simulink model "ScpAp_SafetyModeManager"  (R2025b)
settings: Solver=FixedStepDiscrete  StartTime=0.0  StopTime=10.0  FixedStep=0.02  RelTol=1e-3
undefined symbols (not defined in the file): SafetyMode_L2p_IDT, VechSafetyStatus_L2p_IDT
settings Model: DataDictionary=EgasPOC.sldd  Creator=IAST283  LastModifiedBy=IAST283
settings DataIOCC: SaveFormat=StructureWithTime
settings OptimizationCC: DefaultParameterBehavior=Inlined  EnhancedBackFolding=on  PassReuseOutputArgsAs=Individual arguments  ZeroExternalMemoryAtStartup=off  ZeroInternalMemoryAtStartup=off  OptimizeBlockOrder=speed  DifferentSizesBufferReuse=on  OptimizationCustomize=off  EfficientTunableParamExpr=on
settings DebuggingCC: ParameterTunabilityLossMsg=error
settings SFSimCC: MATLABDynamicMemAlloc=off
settings RTWCC: SystemTargetFile=autosar.tlc  GenCodeOnly=on  TemplateMakefile=ert_default_tmf  DataTypeReplacement=CDataTypesFixedWidth  Description=AUTOSAR
settings CodeAppCC: ForceParamTrailComments=on  IgnoreCustomStorageClasses=off  OperatorAnnotations=on  SimulinkDataObjDesc=on  SFDataObjDesc=on  InsertBlockDesc=on
settings STFCustomTargetCC: SystemTargetFile=autosar.tlc  TargetLangStandard=C99 (ISO)  MultiwordLength=256.0  ParMdlRefBuildCompliant=on  CompOptLevelCompliant=on  ConcurrentExecutionCompliant=off  IncludeMdlTerminateFcn=off  CombineOutputUpdateFcns=on  SuppressErrorStatus=on  ERTCustomFileBanners=on  SupportNonFinite=off  SupportComplex=off  SupportContinuousTime=off  SupportNonInlinedSFcns=off  RemoveResetFunc=on  MATLABClassNameForMDSCustomization=Simulink.SoftwareTarget.ERTCustomization  AutosarCompliant=on  GRTInterface=off  UseToolchainInfoCompliant=on  LookupTableObjectStructAxisOrder=2,1,3,4,...  LUTObjectStructOrderEvenSpacing=Size,Table,Breakpoints  AutosarMatrixIOAsArray=off  AutosarSchemaVersion=R20-11  AutosarCompilerAbstraction=off  DisableAUTOSARRoutinesHostLibrary=off  AutosarMaxShortNameLength=128.0
settings ERTTargetCC: ERTCustomFileTemplate=example_file_process.tlc  BooleanTrueId=TRUE  BooleanFalseId=FALSE  TargetLangStandard=C99 (ISO)  ConcurrentExecutionCompliant=off  IncludeMdlTerminateFcn=off  SuppressErrorStatus=on  SupportNonFinite=off  SupportComplex=off  ModelStepFunctionPrototypeControlCompliant=off  CPPClassGenCompliant=off  AutosarCompliant=on  LookupTableObjectStructAxisOrder=2,1,3,4,...  LUTObjectStructOrderEvenSpacing=Size,Table,Breakpoints

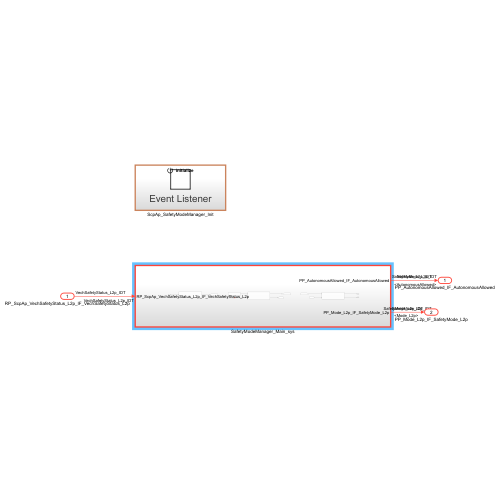
[thumbnail: Simulink's stored preview of the top-level diagram]
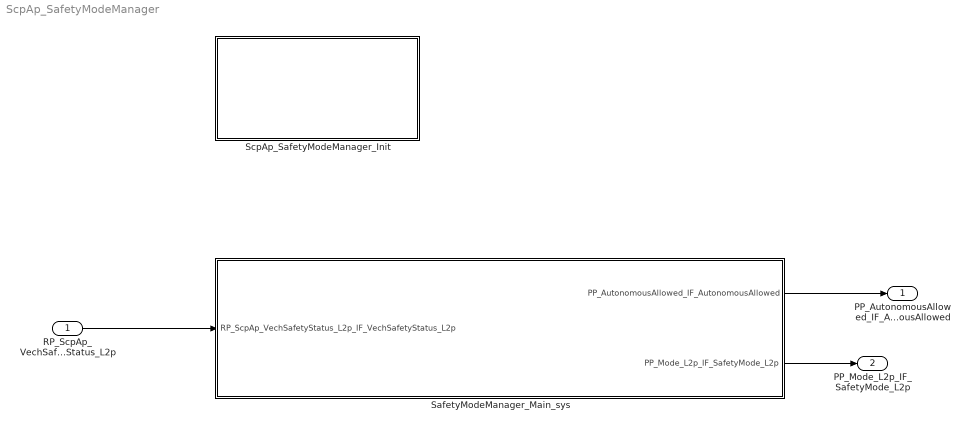
== system ScpAp_SafetyModeManager ==
  RP_ScpAp_VechSafetyStatus_L2p_IF_VechSafetyStatus_L2p : Inport  OutDataTypeStr=Enum: VechSafetyStatus_L2p_IDT  PortDimensions=1
  SafetyModeManager_Main_sys : Subsystem  TreatAsAtomicUnit=on  SystemSampleTime=0.02
  ScpAp_SafetyModeManager_Init : Subsystem
  PP_AutonomousAllowed_IF_AutonomousAllowed : Outport  OutDataTypeStr=Enum: SafetyMode_L2p_IDT  PortDimensions=1
  PP_Mode_L2p_IF_SafetyMode_L2p : Outport  Port=2  OutDataTypeStr=Enum: SafetyMode_L2p_IDT  PortDimensions=1
  wires:
  SafetyModeManager_Main_sys/1(PP_AutonomousAllowed_IF_AutonomousAllowed) -> PP_AutonomousAllowed_IF_AutonomousAllowed/1
  SafetyModeManager_Main_sys/2(PP_Mode_L2p_IF_SafetyMode_L2p) -> PP_Mode_L2p_IF_SafetyMode_L2p/1
  RP_ScpAp_VechSafetyStatus_L2p_IF_VechSafetyStatus_L2p/1 -> SafetyModeManager_Main_sys/1(RP_ScpAp_VechSafetyStatus_L2p_IF_VechSafetyStatus_L2p)

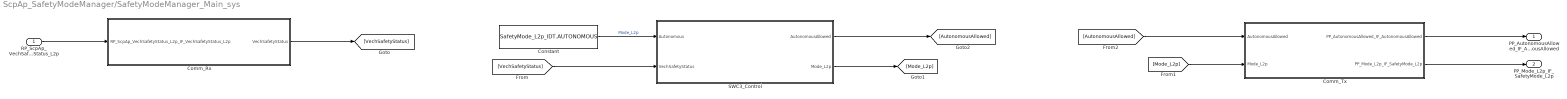
== system ScpAp_SafetyModeManager/SafetyModeManager_Main_sys ==
  RP_ScpAp_VechSafetyStatus_L2p_IF_VechSafetyStatus_L2p : Inport  OutDataTypeStr=Enum: VechSafetyStatus_L2p_IDT  PortDimensions=1
  Comm_Rx : Subsystem
  Comm_Tx : Subsystem
  Constant : Constant  Value=SafetyMode_L2p_IDT.AUTONOMOUS
  SWC3_Control : Subsystem  TreatAsAtomicUnit=on
  PP_AutonomousAllowed_IF_AutonomousAllowed : Outport
  PP_Mode_L2p_IF_SafetyMode_L2p : Outport  Port=2
  wires:
  RP_ScpAp_VechSafetyStatus_L2p_IF_VechSafetyStatus_L2p/1 -> Comm_Rx/1(RP_ScpAp_VechSafetyStatus_L2p_IF_VechSafetyStatus_L2p)
  Comm_Rx/1(VechSafetyStatus) -> [VechSafetyStatus]
  SWC3_Control/1(AutonomousAllowed) -> [AutonomousAllowed]
  [Mode_L2p] -> Comm_Tx/2(Mode_L2p)
  [AutonomousAllowed] -> Comm_Tx/1(AutonomousAllowed)
  Comm_Tx/1(PP_AutonomousAllowed_IF_AutonomousAllowed) -> PP_AutonomousAllowed_IF_AutonomousAllowed/1
  Comm_Tx/2(PP_Mode_L2p_IF_SafetyMode_L2p) -> PP_Mode_L2p_IF_SafetyMode_L2p/1
  Constant/1 -> SWC3_Control/1(Autonomous)  "Mode_L2p"
  [VechSafetyStatus] -> SWC3_Control/2(VechSafetyStatus)
  SWC3_Control/2(Mode_L2p) -> [Mode_L2p]

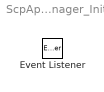
== system ScpAp_SafetyModeManager/ScpAp_SafetyModeManager_Init ==
  Event Listener : EventListener  EventName=reset

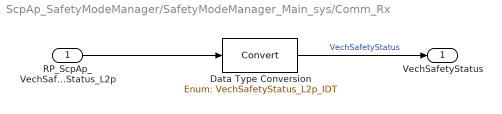
== system ScpAp_SafetyModeManager/SafetyModeManager_Main_sys/Comm_Rx ==
  RP_ScpAp_VechSafetyStatus_L2p_IF_VechSafetyStatus_L2p : Inport  OutDataTypeStr=Enum: VechSafetyStatus_L2p_IDT
  Data Type Conversion : DataTypeConversion  OutDataTypeStr=Enum: VechSafetyStatus_L2p_IDT  SaturateOnIntegerOverflow=off  RndMeth=Floor
  VechSafetyStatus : Outport
  wires:
  RP_ScpAp_VechSafetyStatus_L2p_IF_VechSafetyStatus_L2p/1 -> Data Type Conversion/1
  Data Type Conversion/1 -> VechSafetyStatus/1  "VechSafetyStatus"

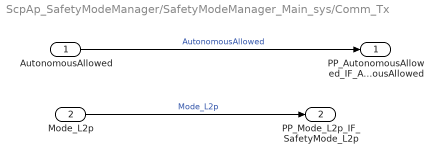
== system ScpAp_SafetyModeManager/SafetyModeManager_Main_sys/Comm_Tx ==
  AutonomousAllowed : Inport  OutDataTypeStr=Enum: SafetyMode_L2p_IDT
  Mode_L2p : Inport  Port=2
  PP_AutonomousAllowed_IF_AutonomousAllowed : Outport  OutDataTypeStr=Enum: SafetyMode_L2p_IDT
  PP_Mode_L2p_IF_SafetyMode_L2p : Outport  Port=2
  wires:
  Mode_L2p/1 -> PP_Mode_L2p_IF_SafetyMode_L2p/1  "Mode_L2p"
  AutonomousAllowed/1 -> PP_AutonomousAllowed_IF_AutonomousAllowed/1  "AutonomousAllowed"

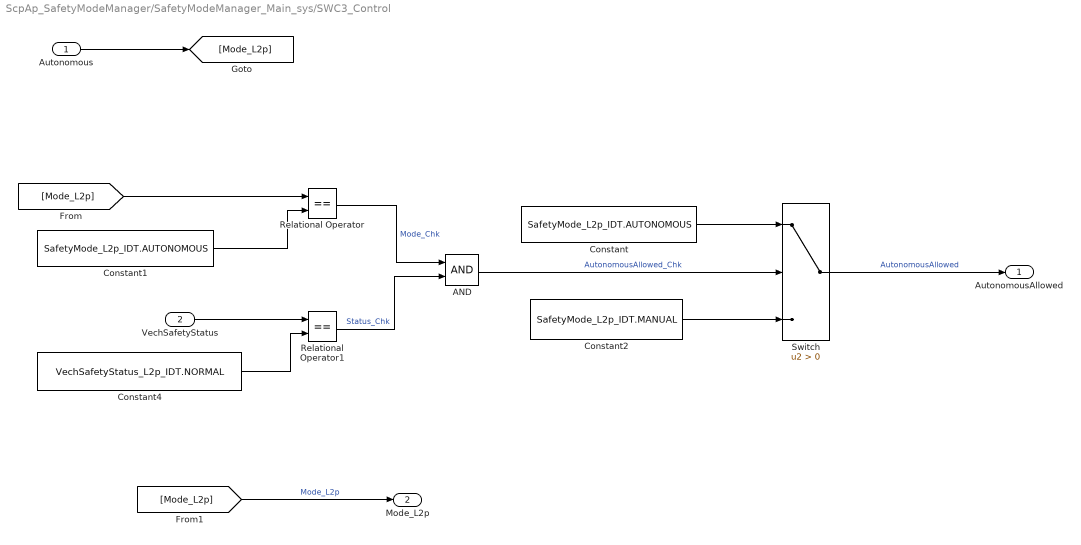
== system ScpAp_SafetyModeManager/SafetyModeManager_Main_sys/SWC3_Control ==
  Autonomous : Inport
  VechSafetyStatus : Inport  Port=2  OutDataTypeStr=Enum: VechSafetyStatus_L2p_IDT
  AND : Logic  AllPortsSameDT=off  OutDataTypeStr=boolean
  Constant : Constant  Value=SafetyMode_L2p_IDT.AUTONOMOUS  OutDataTypeStr=Enum: SafetyMode_L2p_IDT
  Constant1 : Constant  Value=SafetyMode_L2p_IDT.AUTONOMOUS  OutDataTypeStr=Enum: SafetyMode_L2p_IDT
  Constant2 : Constant  Value=SafetyMode_L2p_IDT.MANUAL  OutDataTypeStr=Enum: SafetyMode_L2p_IDT
  Constant4 : Constant  Value=VechSafetyStatus_L2p_IDT.NORMAL  OutDataTypeStr=Enum: VechSafetyStatus_L2p_IDT
  Relational Operator : RelationalOperator  Operator===  OutDataTypeStr=boolean  RndMeth=Simplest  InputSameDT=off
  Relational Operator1 : RelationalOperator  Operator===  OutDataTypeStr=boolean  RndMeth=Simplest  InputSameDT=off
  Switch : Switch  Criteria=u2 > Threshold  SaturateOnIntegerOverflow=off  InputSameDT=off
  AutonomousAllowed : Outport  OutDataTypeStr=Enum: SafetyMode_L2p_IDT
  Mode_L2p : Outport  Port=2
  wires:
  Constant1/1 -> Relational Operator/2
  Relational Operator/1 -> AND/1  "Mode_Chk"
  AND/1 -> Switch/2  "AutonomousAllowed_Chk"
  Constant4/1 -> Relational Operator1/2
  Relational Operator1/1 -> AND/2  "Status_Chk"
  Autonomous/1 -> [Mode_L2p]
  [Mode_L2p] -> Mode_L2p/1  "Mode_L2p"
  Switch/1 -> AutonomousAllowed/1  "AutonomousAllowed"
  Constant/1 -> Switch/1
  Constant2/1 -> Switch/3
  [Mode_L2p] -> Relational Operator/1
  VechSafetyStatus/1 -> Relational Operator1/1
